simulink model "pe_pmsm_drive_project"  (R2018b)
settings: Solver=VariableStepAuto  StartTime=0.0  StopTime=0.5  FixedStep=1e-3  MaxStep=2.0E-6  RelTol=1e-6  AbsTol=1e-3  EnableMultiTasking=on
PreLoadFcn:
  | % Control parameters
  | Ts = 2e-6;   % Fundamental sample time
  | fsw = 2e3;   % Switching frequency (Hz)
  | fc = fsw*10; % Control loop frequency (Hz)
  | Tsc = 1/fc;  % Control loop sample time
  | 
  | % PMSM parameters
  | PM = 0.03; % Permanent magnet flux linkage
  | Ld = 2e-4;  % d-axis inductance
  | Lq = 2e-4;  % q-axis inductance
  | L0 = 2e-4;  % 0-axis inductance
  | Rs = 0.013; % Stator resistance
  | N = 6; % Number of pole pairs
  | J = 0.2; % Moment of inertia
  | 
  | % Operating and derived limits
  | Imax = 100;  % Max stator current (peak value)
  | Tmax = 1.5*N*PM*Imax; % Max lectromagnetic torque
  | fnom = 100;  % Nominal frequency (Hz)
  | rpm_nom = 60*fnom/N;      % Nominal rotor speed (rpm)
  | omegam_nom = 2*pi*fnom/N; % Nominal mechanical rotor speed
  | Pmax = omegam_nom*Tmax;     % Maximum power
values from neighbouring files (symbols this model uses):
  faero = 0.5*cd*frontarea*airdens.*speed.^2    [PMSM.m]    (also in PMSM_trqlimiter.m)
  rt = 3    [PMSM.m]    (also in PMSM_trqlimiter.m)
  speed = linspace(0, 60, 1000)    [PMSM.m]    (also in PMSM_trqlimiter.m)
  wheelrad = 0.3    [PMSM.m]    (also in PMSM_trqlimiter.m)
libraries: nesl_utility x12, pe_lib x10, fl_lib x8, pePmsmFieldOrientedControl x1, simulink x1
CloseFcn:
  | try
  |   clear Imax J L0 Ld Lq N PM Pmax Rs
  |   clear Tmax Ts Tsc fc fnom fsw
  |   clear omegam_nom rpm_nom tout
  | end
Description:
  | Three-Phase PMSM Drive
  | 
  | This example shows a Permanent Magnet Synchronous Machine
  | (PMSM) and inverter sized for use in a typical hybrid vehicle.
  | Here the inverter is connected directly to the vehicle battery, but
  | often there is also a DC-DC converter stage in between. The
  | model can be used to design the PMSM controller, selecting
  | architecture and gains to achieve desired performance. To check
  | the timing of IGBT turn-on and turn-off, the IGBT devices can be
  | directly replaced by more detailed device models from
  | Simscape(TM) Electronics(TM). For complete vehicle modeling, the
  | Simscape Electronics Servomotor block can be used to abstract
  | the PMSM, inverter and controller with an energy-based model.
  | The Gmin resistor provides a very small conductance to ground
  | that improves the numerical properties of the model when using
  | a variable-step solver.
  | 
  | Copyright 2014-2017 The MathWorks, Inc.
settings Model: Creator=The MathWorks, Inc.  LastModifiedBy=Giorgia
settings SolverCC: AutoScaleAbsTol=off  MaxConsecutiveMinStep=2
settings DataIOCC: LimitDataPoints=on  SaveFormat=Array
settings OptimizationCC: LifeSpan=inf
settings DebuggingCC: UnderspecifiedInitializationDetection=Classic  MergeDetectMultiDrivingBlocksExec=none  MaxConsecutiveZCsMsg=none  AllowSymbolicDim=off  LibraryContextMissingDiagnostic=none  SFUnexpectedBacktrackingDiag=warning  SFNoUnconditionalDefaultTransitionDiag=warning  SFExecutionAtInitializationDiag=none
settings HardwareCC: ProdBitPerPointer=32  ProdBitPerSizeT=32  ProdBitPerPtrDiffT=32  ProdLargestAtomicFloat=None  ProdIntDivRoundTo=Undefined  ProdEndianess=Unspecified  ProdWordSize=32  ProdHWDeviceType=32-bit Generic
settings ModelReferenceCC: PropagateSignalLabelsOutOfModel=off
settings SFSimCC: SimUseLocalCustomCode=off
settings RTWCC: RTWUseLocalCustomCode=off
settings CodeAppCC: StateflowObjectComments=on
settings GRTTargetCC: TargetLangStandard=C89/C90 (ANSI)  GeneratePreprocessorConditionals=Disable all
settings ConfigComp: CovMetricSettings=dw  CovHtmlReporting=on  CovSaveCumulativeToWorkspaceVar=on  CovSaveSingleToWorkspaceVar=on  CovShowResultsExplorer=off  CovExternalEMLEnable=off  CovSFcnEnable=off

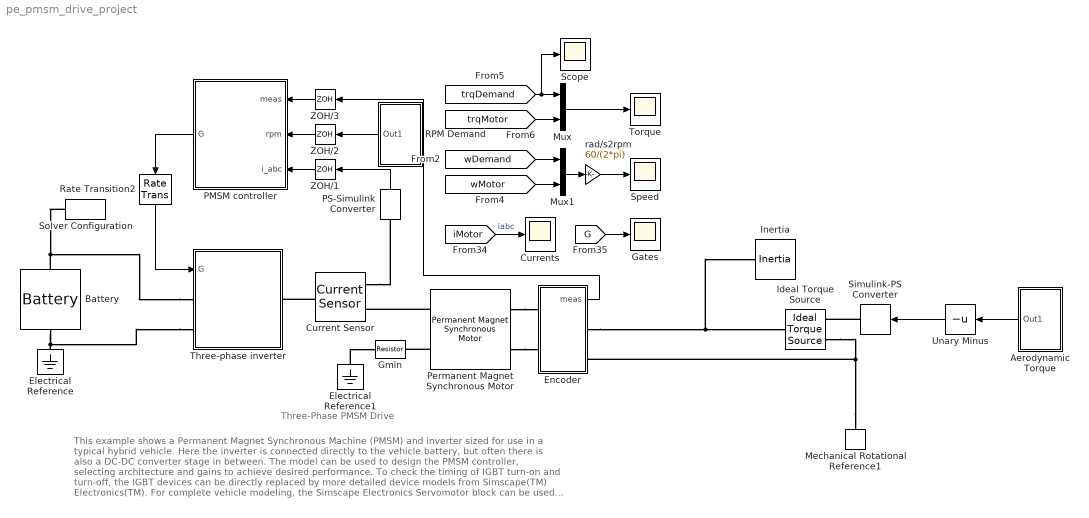
== system pe_pmsm_drive_project ==
  note: This example shows a Permanent Magnet Synchronous Machine (PMSM) and inverter sized for use in a typical hybrid vehicle.
      | Here the inverter is connected directly to the vehicle battery, but often there is also a DC-DC converter stage in between. The
      | model can be used to design the PMSM controller, selecting architecture and gains to achieve desired performance. To check
      | the timing of IGBT turn-on and turn-off, the IGBT devices can be directly replaced by more detailed device models from
      | Simscape(TM) Electronics(TM). For complete vehicle modeling, the Simscape Electronics Servomotor block can be used to
      | abstract the PMSM, inverter and controller with an energy-based model. The Gmin resistor provides a very small conductance
      | to ground that improves the numerical properties of the model when using a variable-step solver.
  note: Three-Phase PMSM Drive
  Aerodynamic Torque : Subsystem
  Battery : pe_lib/Sources/Battery  Vnom=110 V  R1=0.001 Ohm  prm_AH=1  AH=14000 hr*A  V1=470 V  AH1=5000 hr*A  prm_R2=1  R2=inf Ohm  prm_dyn=1  Rp1=0.005 Ohm  tau1=30 s  Rp2=0.005 Ohm  tau2=30 s  Rp3=0.005 Ohm  tau3=30 s  Rp4=0.005 Ohm  tau4=30 s  Rp5=0.005 Ohm  tau5=30 s  prm_fade=1  N_fade=100  AH_fade=45 hr*A  R1_fade=2.02 Ohm  V1_fade=10.35 V  i_specify=off  i_priority=None  i=0 A  i_nominal_specify=off  i_nominal_unit=A  i_nominal_value=1  v_specify=off  v_priority=None  v=0 V  v_nominal_specify=off  v_nominal_unit=V  v_nominal_value=1  charge_specify=on  charge_priority=High  charge=7000 hr*A  charge_nominal_specify=off  charge_nominal_unit=hr*A  charge_nominal_value=1  num_cycles_specify=off  num_cycles_priority=High  num_cycles=0  num_cycles_nominal_specify=off  num_cycles_nominal_unit=1  num_cycles_nominal_value=1  thermal_mass=30000 J/K  Tmeas=298.15 K  Vnom_T2=12 V  R1_T2=2.2 Ohm  V1_T2=11.4 V  R2_T2=2200 Ohm  Rp1_T2=0.005 Ohm  tau1_T2=30 s  Rp2_T2=0.005 Ohm  tau2_T2=30 s  Rp3_T2=0.005 Ohm  tau3_T2=30 s  Rp4_T2=0.005 Ohm  tau4_T2=30 s  Rp5_T2=0.005 Ohm  tau5_T2=30 s  Tmeas2=273.15 K  temperature_specify=off  temperature_priority=High  temperature=298.15 K  temperature_nominal_specify=off  temperature_nominal_unit=K  temperature_nominal_value=1
      settings: SourceProductName=Simscape Electrical  SourceProductBaseCode=PS
  Current Sensor : pe_lib/Sensors/Current Sensor
      settings: SourceProductName=Simscape Electrical  SourceProductBaseCode=PS
  Currents : Scope
  Electrical Reference : fl_lib/Electrical/Electrical Elements/Electrical Reference
      settings: SourceProductName=Foundation Library
  Electrical Reference1 : fl_lib/Electrical/Electrical Elements/Electrical Reference
      settings: SourceProductName=Foundation Library
  Encoder : Subsystem
  Gates : Scope
  Gmin : fl_lib/Electrical/Electrical Elements/Resistor  R=1e9 Ohm  i_specify=off  i_priority=High  i=0 A  i_nominal_specify=off  i_nominal_unit=A  i_nominal_value=1  v_specify=off  v_priority=High  v=0 V  v_nominal_specify=off  v_nominal_unit=V  v_nominal_value=1
      settings: SourceProductName=Foundation Library
  Ideal Torque Source : fl_lib/Mechanical/Mechanical Sources/Ideal Torque Source
  Inertia : fl_lib/Mechanical/Rotational Elements/Inertia  inertia=0.01 kg*m^2  w_specify=off  w_priority=High  w=0 rad/s  w_nominal_specify=off  w_nominal_unit=rad/s  w_nominal_value=1  t_specify=off  t_priority=None  t=0 N*m  t_nominal_specify=off  t_nominal_unit=N*m  t_nominal_value=1
  Mechanical Rotational Reference1 : fl_lib/Mechanical/Rotational Elements/Mechanical Rotational Reference
      settings: SourceProductName=Foundation Library
  Mux : Mux  Inputs=2
  Mux1 : Mux  Inputs=2
  PMSM controller : Subsystem
  PS-Simulink Converter : nesl_utility/PS-Simulink Converter  PhysicalDomain=network_engine_domain  SubClassName=ps_output  LeftPortType=input  RightPortType=output  PseudoPeriodic=off  Frequencies=[]  Unit=A  AffineConversion=off
  Permanent Magnet Synchronous Motor : pe_lib/Machines/Permanent Magnet Rotor/Permanent Magnet Synchronous Motor  nPolePairs=N  pmflux_param=1  pm_flux_linkage=PM Wb  torque_constant=0.18 N*m/A  back_emf_constant=0.18 V/(rad/s)  stator_param=1  Ld=Ld H  Lq=Lq H  L0=L0 H  Ls=0.0002 H  Lm=0.00002 H  Ms=0.00002 H  Rs=Rs Ohm  zero_sequence=pe.enum.park.zerosequence.include  J=0 kg*m^2  lam=0 N*m/(rad/s)  axes_param=1  i_d_specify=off  i_d_priority=None  i_d=0 A  i_d_nominal_specify=off  i_d_nominal_unit=A  i_d_nominal_value=1  i_q_specify=off  i_q_priority=None  i_q=0 A  i_q_nominal_specify=off  i_q_nominal_unit=A  i_q_nominal_value=1  torque_specify=off  torque_priority=None  torque=0 N*m  torque_nominal_specify=off  torque_nominal_unit=N*m  torque_nominal_value=1  angular_velocity_specify=on  angular_velocity_priority=None  angular_velocity=0 rpm  angular_velocity_nominal_specify=off  angular_velocity_nominal_unit=rpm  angular_velocity_nominal_value=1  angular_position_specify=on  angular_position_priority=High  angular_position=0 rad  angular_position_nominal_specify=off  angular_position_nominal_unit=deg  angular_position_nominal_value=1
      settings: SourceProductName=Simscape Electrical  SourceProductBaseCode=PS
  RPM Demand : Subsystem
  Rate Transition2 : RateTransition  OutPortSampleTime=Ts
  Scope : Scope
  Simulink-PS Converter : nesl_utility/Simulink-PS Converter  PhysicalDomain=network_engine_domain  SubClassName=ps_input  LeftPortType=input  RightPortType=output  PseudoPeriodic=off  Frequencies=[]  NoiseDistribution=none  NoiseParameters=[]  Unit=1  AffineConversion=off  FilteringAndDerivatives=provide  SimscapeFilterOrder=1  InputFilterTimeConstant=0.001  UdotUserProvided=0
  Solver Configuration : nesl_utility/Solver Configuration  PhysicalDomain=network_engine_domain  SubClassName=solver  LeftPortType=input  RightPortType=generic  Tones=[]  Harmonics=[]  SimulateNoise=off  Profile=off  UseLocalSampling=off  EnableSwitchedLinearOptims=on  FrequencyDomain=off  UseCCode=off  RelTol=0.001  AbsTol=1e-06  MinStep=1e-09  ToWorkspace=off  RevertToSquareIcSolve=off  NumHomotopyIterations=100  PhasorMode=off  PhasorModeNumHarmonics=1  DoDC=off  ResidualTolerance=1e-9  UseLocalSolver=on  LocalSolverChoice=NE_BACKWARD_EULER_ADVANCER  LocalSolverSampleTime=Ts  DoFixedCost=on  MaxNonlinIter=4  MaxModeIter=2  LinearAlgebra=Sparse  EquationFormulation=NE_TIME_EF  DelaysMemoryBudget=1024  AutomaticFiltering=on  FilteringTimeConstant=0.001  PartitionStorageMethod=AS_NEEDED  PartitionMemoryBudget=1024
  Speed : Scope
  Three-phase inverter : Subsystem
  Torque : Scope
  Unary Minus : UnaryMinus
  ZOH/1 : ZeroOrderHold  SampleTime=Tsc
  ZOH/2 : ZeroOrderHold  SampleTime=Tsc
  ZOH/3 : ZeroOrderHold  SampleTime=Tsc
  rad/s2rpm : Gain  Gain=60/(2*pi)
  wires:
  RPM Demand/1(Out1) -> ZOH/2/1
  PS-Simulink Converter/1 -> ZOH/1/1
  Mux1/1 -> rad/s2rpm/1
  [iMotor] -> Currents/1  "iabc"
  [G] -> Gates/1
  [wDemand] -> Mux1/1
  Mux/1 -> Torque/1
  [trqMotor] -> Mux/2
  [trqDemand] -> Scope/1, Mux/1
  Encoder/1(meas) -> ZOH/3/1
  ZOH/3/1 -> PMSM controller/1(meas)
  ZOH/2/1 -> PMSM controller/2(rpm)
  ZOH/1/1 -> PMSM controller/3(i_abc)
  Rate Transition2/1 -> Three-phase inverter/1(G)
  [wMotor] -> Mux1/2
  rad/s2rpm/1 -> Speed/1
  PMSM controller/1(G) -> Rate Transition2/1
  Aerodynamic Torque/1(Out1) -> Unary Minus/1
  Unary Minus/1 -> Simulink-PS Converter/1
  connections:
  Three-phase inverter/LConn1 -- Solver Configuration/RConn1 -- Battery/LConn1
  Permanent Magnet Synchronous Motor/RConn1 -- Encoder/LConn1
  Permanent Magnet Synchronous Motor/RConn2 -- Encoder/LConn2
  Current Sensor/LConn1 -- Three-phase inverter/RConn1
  Three-phase inverter/LConn2 -- Electrical Reference/LConn1 -- Battery/RConn1
  Permanent Magnet Synchronous Motor/LConn1 -- Current Sensor/RConn2
  Current Sensor/RConn1 -- PS-Simulink Converter/LConn1
  Permanent Magnet Synchronous Motor/LConn2 -- Gmin/RConn1
  Electrical Reference1/LConn1 -- Gmin/LConn1
  Encoder/RConn1 -- Ideal Torque Source/LConn1 -- Inertia/LConn1
  Mechanical Rotational Reference1/LConn1 -- Encoder/RConn2 -- Ideal Torque Source/RConn2
  Simulink-PS Converter/RConn1 -- Ideal Torque Source/RConn1

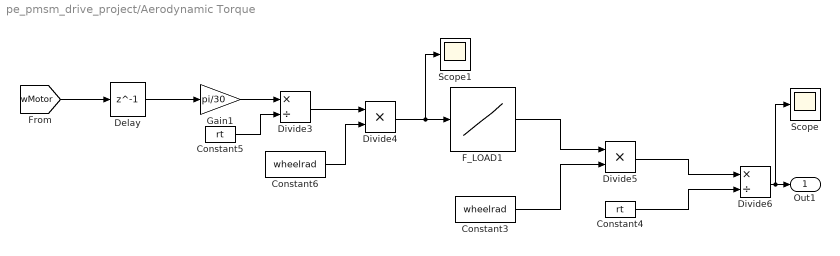
== system pe_pmsm_drive_project/Aerodynamic Torque ==
  Constant3 : Constant  Value=wheelrad
  Constant4 : Constant  Value=rt
  Constant5 : Constant  Value=rt
  Constant6 : Constant  Value=wheelrad
  Delay : Delay  DelayLength=1  InitialCondition=0
  Divide3 : Product  Inputs=*/
  Divide4 : Product  Inputs=**
  Divide5 : Product  Inputs=**
  Divide6 : Product  Inputs=*/
  F_LOAD1 : Lookup_n-D  NumberOfTableDimensions=1  BreakpointsForDimension1=speed  Table=faero  ExtrapMethod=Clip  UseLastTableValue=on  InternalRulePriority=Speed  RndMeth=Simplest  InputSameDT=on
  Gain1 : Gain  Gain=pi/30
  Scope : Scope
  Scope1 : Scope
  Out1 : Outport
  wires:
  F_LOAD1/1 -> Divide5/1
  Constant3/1 -> Divide5/2
  Divide5/1 -> Divide6/1
  Constant4/1 -> Divide6/2
  Divide6/1 -> Scope/1, Out1/1
  Constant5/1 -> Divide3/2
  Gain1/1 -> Divide3/1
  Divide3/1 -> Divide4/1
  Constant6/1 -> Divide4/2
  Divide4/1 -> Scope1/1, F_LOAD1/1
  [wMotor] -> Delay/1
  Delay/1 -> Gain1/1

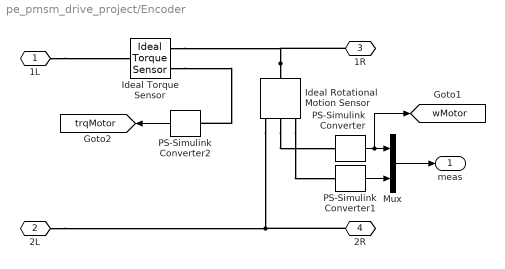
== system pe_pmsm_drive_project/Encoder ==
  Ideal Rotational Motion Sensor : fl_lib/Mechanical/Mechanical Sensors/Ideal Rotational Motion Sensor  offset=0 deg
      settings: SourceProductName=Foundation Library
  Ideal Torque Sensor : fl_lib/Mechanical/Mechanical Sensors/Ideal Torque Sensor
      settings: SourceProductName=Foundation Library
  Mux : Mux  Inputs=2
  PS-Simulink Converter : nesl_utility/PS-Simulink Converter  PhysicalDomain=network_engine_domain  SubClassName=ps_output  LeftPortType=input  RightPortType=output  PseudoPeriodic=off  Frequencies=[]  Unit=rad/s  AffineConversion=off
  PS-Simulink Converter1 : nesl_utility/PS-Simulink Converter  PhysicalDomain=network_engine_domain  SubClassName=ps_output  LeftPortType=input  RightPortType=output  PseudoPeriodic=off  Frequencies=[]  Unit=rad  AffineConversion=off
  PS-Simulink Converter2 : nesl_utility/PS-Simulink Converter  PhysicalDomain=network_engine_domain  SubClassName=ps_output  LeftPortType=input  RightPortType=output  PseudoPeriodic=off  Frequencies=[]  Unit=N*m  AffineConversion=off
  1L : PMIOPort  Side=Left
  2L : PMIOPort  Port=2  Side=Left
  1R : PMIOPort  Port=3  Side=Right
  2R : PMIOPort  Port=4  Side=Right
  meas : Outport
  tag scope: trqMotor=global, wMotor=global
  wires:
  PS-Simulink Converter2/1 -> [trqMotor]
  Mux/1 -> meas/1
  PS-Simulink Converter1/1 -> Mux/2
  PS-Simulink Converter/1 -> [wMotor], Mux/1
  connections:
  Ideal Torque Sensor/RConn2 -- PS-Simulink Converter2/LConn1
  1L/RConn1 -- Ideal Torque Sensor/LConn1
  2R/RConn1 -- 2L/RConn1 -- Ideal Rotational Motion Sensor/RConn1
  Ideal Rotational Motion Sensor/LConn1 -- 1R/RConn1 -- Ideal Torque Sensor/RConn1
  Ideal Rotational Motion Sensor/RConn2 -- PS-Simulink Converter/LConn1
  Ideal Rotational Motion Sensor/RConn3 -- PS-Simulink Converter1/LConn1

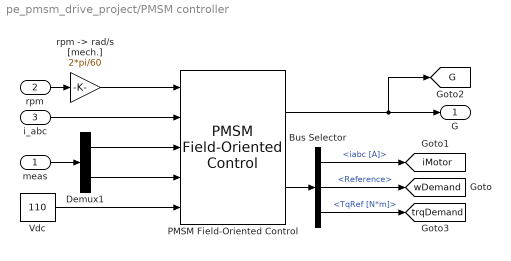
== system pe_pmsm_drive_project/PMSM controller ==
  meas : Inport
  rpm : Inport  Port=2
  i_abc : Inport  Port=3
  Bus Selector : BusSelector  OutputSignals=iabc [A],Reference,TqRef [N*m]
  Demux1 : Demux  Outputs=2
  PMSM Field-Oriented Control : pePmsmFieldOrientedControl/PMSM Field-Oriented Control  CtrlMode=Velocity control  Vnom=110  Pmax=Pmax  Tmax=Tmax*1.5  p=N  Vdc_on=10  Ts=Ts  Tsc=Tsc  CtrlType=PI control  Kp_w=6  Ki_w=200  Kv_w=1  Kaw_w=1000  RefType=Zero d-axis control  rpmVec=[0, 3000]  TqVec=[-100, 0, 100]  VdcVec=[300, 350]  idMatrix=zeros(2,3,2)  iqMatrix=zeros(2,3,2)  psim=PM  Ld=0.00024  Lq=0.00029  Rs=0.01  AxisAlignment=Q-axis  Kp_id=0.1  Ki_id=10  Kaw_id=1000  Kp_iq=0.1  Ki_iq=10  Kaw_iq=1000  AxisPrio=Q-axis  ActZC=off  ActFF=on  ParamTypeFF=Constant parameters  LdFF=Ld  LqFF=Lq  psimFF=PM  idVect=[-200, 0, 200]  iqVect=[-200, 0, 200]  LdMatrix=0.0002 * ones(3, 3)  LqMatrix=0.0002 * ones(3, 3)  psimMatrix=0.04 * ones(3, 3)  CPWMMode=SPWM: sinusoidal PWM  fsw=fsw
      settings: SamplingMode=Natural
  Vdc : Constant  Value=110  SampleTime=Tsc
  "rpm -> rad/s [mech.]" : Gain  Gain=2*pi/60
  G : Outport
  tag scope: G=global, iMotor=global, trqDemand=global, wDemand=global
  wires:
  PMSM Field-Oriented Control/1 -> G/1, [G]
  Vdc/1 -> PMSM Field-Oriented Control/5
  PMSM Field-Oriented Control/2 -> Bus Selector/1
  i_abc/1 -> PMSM Field-Oriented Control/2
  meas/1 -> Demux1/1
  Demux1/1 -> PMSM Field-Oriented Control/3
  Demux1/2 -> PMSM Field-Oriented Control/4
  Bus Selector/1 -> [iMotor]  "<iabc [A]>"
  Bus Selector/2 -> [wDemand]  "<Reference>"
  Bus Selector/3 -> [trqDemand]  "<TqRef [N*m]>"
  rpm/1 -> "rpm -> rad/s [mech.]"/1
  "rpm -> rad/s [mech.]"/1 -> PMSM Field-Oriented Control/1

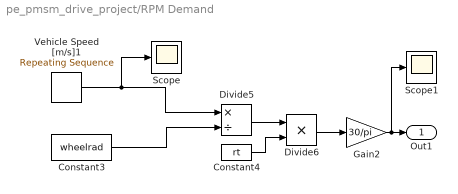
== system pe_pmsm_drive_project/RPM Demand ==
  Constant3 : Constant  Value=wheelrad
  Constant4 : Constant  Value=rt
  Divide5 : Product  Inputs=*/
  Divide6 : Product  Inputs=**
  Gain2 : Gain  Gain=30/pi
  Scope : Scope
  Scope1 : Scope
  Vehicle Speed [m/s]1 : simulink/Sources/Repeating Sequence  rep_seq_t=time  rep_seq_y=vehiclespeed
  Out1 : Outport
  wires:
  Vehicle Speed [m/s]1/1 -> Scope/1, Divide5/1
  Constant4/1 -> Divide6/2
  Divide6/1 -> Gain2/1
  Divide5/1 -> Divide6/1
  Constant3/1 -> Divide5/2
  Gain2/1 -> Scope1/1, Out1/1

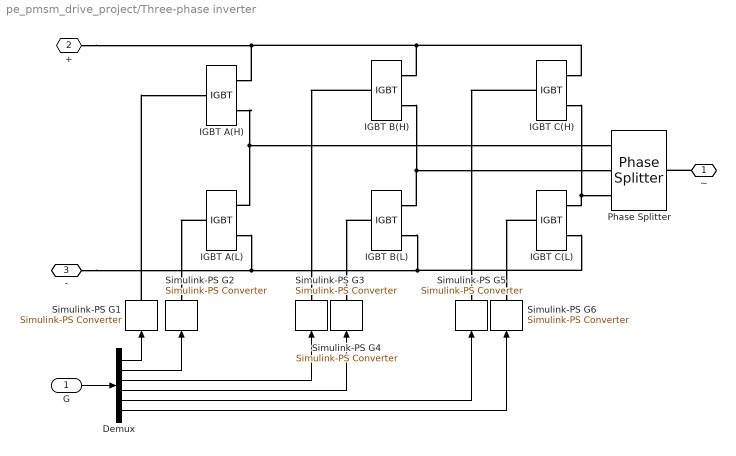
== system pe_pmsm_drive_project/Three-phase inverter ==
  G : Inport
  Demux : Demux  Outputs=6
  IGBT A(H) : pe_lib/Semiconductors/Fundamental Components/IGBT  Vf=0.8 V  Ron=0.001 Ohm  Goff=1e-5 S  Vth=0.5 V  diode_param=2  diode_Vf=0.8 V  diode_Ron=0.001 Ohm  diode_Goff=1e-5 S  diode_C=5e-8 F  diode_iRM=-235 A  diode_iF=300 A  diode_idot=-50 A/us  diode_trr_param=1  diode_trr_factor=3  diode_trr=15 us  diode_Qrr=1.5e+3 s*uA  thermal_loss_option=1  Voff=300 V  Tau=0.1 s  Tj=[ 298.15 398.15 ] K  Iout_scalar=600 A  Eon_scalar=0.02286 J  Eoff_scalar=0.01714 J  Von_scalar=2.7 V  Iout_data=[ 0 10 50 100 200 400 600 ] A  Eon_data=[ 0 2.9e-4 0.00143 0.00286 0.00571 0.01314 0.02286; 0 5.7e-4 0.00263 0.00514 0.01029 0.02057 0.03029 ] J  Eoff_data=[ 0 2.1e-4 0.00107 0.00214 0.00429 0.009859999999999999 0.01714; 0 4.3e-4 0.00197 0.00386 0.00771 0.01543 0.02271 ] J  Von_data=[ 0 1.1 1.3 1.45 1.75 2.25 2.7; 0 1 1.15 1.35 1.7 2.35 3 ] V
      settings: SourceProductName=Simscape Electrical  SourceProductBaseCode=PS
  IGBT A(L) : pe_lib/Semiconductors/Fundamental Components/IGBT  Vf=0.8 V  Ron=0.001 Ohm  Goff=1e-5 S  Vth=0.5 V  diode_param=2  diode_Vf=0.8 V  diode_Ron=0.001 Ohm  diode_Goff=1e-5 S  diode_C=5e-8 F  diode_iRM=-235 A  diode_iF=300 A  diode_idot=-50 A/us  diode_trr_param=1  diode_trr_factor=3  diode_trr=15 us  diode_Qrr=1.5e+3 s*uA  thermal_loss_option=1  Voff=300 V  Tau=0.1 s  Tj=[ 298.15 398.15 ] K  Iout_scalar=600 A  Eon_scalar=0.02286 J  Eoff_scalar=0.01714 J  Von_scalar=2.7 V  Iout_data=[ 0 10 50 100 200 400 600 ] A  Eon_data=[ 0 2.9e-4 0.00143 0.00286 0.00571 0.01314 0.02286; 0 5.7e-4 0.00263 0.00514 0.01029 0.02057 0.03029 ] J  Eoff_data=[ 0 2.1e-4 0.00107 0.00214 0.00429 0.009859999999999999 0.01714; 0 4.3e-4 0.00197 0.00386 0.00771 0.01543 0.02271 ] J  Von_data=[ 0 1.1 1.3 1.45 1.75 2.25 2.7; 0 1 1.15 1.35 1.7 2.35 3 ] V
      settings: SourceProductName=Simscape Electrical  SourceProductBaseCode=PS
  IGBT B(H) : pe_lib/Semiconductors/Fundamental Components/IGBT  Vf=0.8 V  Ron=0.001 Ohm  Goff=1e-5 S  Vth=0.5 V  diode_param=2  diode_Vf=0.8 V  diode_Ron=0.001 Ohm  diode_Goff=1e-5 S  diode_C=5e-8 F  diode_iRM=-235 A  diode_iF=300 A  diode_idot=-50 A/us  diode_trr_param=1  diode_trr_factor=3  diode_trr=15 us  diode_Qrr=1.5e+3 s*uA  thermal_loss_option=1  Voff=300 V  Tau=0.1 s  Tj=[ 298.15 398.15 ] K  Iout_scalar=600 A  Eon_scalar=0.02286 J  Eoff_scalar=0.01714 J  Von_scalar=2.7 V  Iout_data=[ 0 10 50 100 200 400 600 ] A  Eon_data=[ 0 2.9e-4 0.00143 0.00286 0.00571 0.01314 0.02286; 0 5.7e-4 0.00263 0.00514 0.01029 0.02057 0.03029 ] J  Eoff_data=[ 0 2.1e-4 0.00107 0.00214 0.00429 0.009859999999999999 0.01714; 0 4.3e-4 0.00197 0.00386 0.00771 0.01543 0.02271 ] J  Von_data=[ 0 1.1 1.3 1.45 1.75 2.25 2.7; 0 1 1.15 1.35 1.7 2.35 3 ] V
      settings: SourceProductName=Simscape Electrical  SourceProductBaseCode=PS
  IGBT B(L) : pe_lib/Semiconductors/Fundamental Components/IGBT  Vf=0.8 V  Ron=0.001 Ohm  Goff=1e-5 S  Vth=0.5 V  diode_param=2  diode_Vf=0.8 V  diode_Ron=0.001 Ohm  diode_Goff=1e-5 S  diode_C=5e-8 F  diode_iRM=-235 A  diode_iF=300 A  diode_idot=-50 A/us  diode_trr_param=1  diode_trr_factor=3  diode_trr=15 us  diode_Qrr=1.5e+3 s*uA  thermal_loss_option=1  Voff=300 V  Tau=0.1 s  Tj=[ 298.15 398.15 ] K  Iout_scalar=600 A  Eon_scalar=0.02286 J  Eoff_scalar=0.01714 J  Von_scalar=2.7 V  Iout_data=[ 0 10 50 100 200 400 600 ] A  Eon_data=[ 0 2.9e-4 0.00143 0.00286 0.00571 0.01314 0.02286; 0 5.7e-4 0.00263 0.00514 0.01029 0.02057 0.03029 ] J  Eoff_data=[ 0 2.1e-4 0.00107 0.00214 0.00429 0.009859999999999999 0.01714; 0 4.3e-4 0.00197 0.00386 0.00771 0.01543 0.02271 ] J  Von_data=[ 0 1.1 1.3 1.45 1.75 2.25 2.7; 0 1 1.15 1.35 1.7 2.35 3 ] V
      settings: SourceProductName=Simscape Electrical  SourceProductBaseCode=PS
  IGBT C(H) : pe_lib/Semiconductors/Fundamental Components/IGBT  Vf=0.8 V  Ron=0.001 Ohm  Goff=1e-5 S  Vth=0.5 V  diode_param=2  diode_Vf=0.8 V  diode_Ron=0.001 Ohm  diode_Goff=1e-5 S  diode_C=5e-8 F  diode_iRM=-235 A  diode_iF=300 A  diode_idot=-50 A/us  diode_trr_param=1  diode_trr_factor=3  diode_trr=15 us  diode_Qrr=1.5e+3 s*uA  thermal_loss_option=1  Voff=300 V  Tau=0.1 s  Tj=[ 298.15 398.15 ] K  Iout_scalar=600 A  Eon_scalar=0.02286 J  Eoff_scalar=0.01714 J  Von_scalar=2.7 V  Iout_data=[ 0 10 50 100 200 400 600 ] A  Eon_data=[ 0 2.9e-4 0.00143 0.00286 0.00571 0.01314 0.02286; 0 5.7e-4 0.00263 0.00514 0.01029 0.02057 0.03029 ] J  Eoff_data=[ 0 2.1e-4 0.00107 0.00214 0.00429 0.009859999999999999 0.01714; 0 4.3e-4 0.00197 0.00386 0.00771 0.01543 0.02271 ] J  Von_data=[ 0 1.1 1.3 1.45 1.75 2.25 2.7; 0 1 1.15 1.35 1.7 2.35 3 ] V
      settings: SourceProductName=Simscape Electrical  SourceProductBaseCode=PS
  IGBT C(L) : pe_lib/Semiconductors/Fundamental Components/IGBT  Vf=0.8 V  Ron=0.001 Ohm  Goff=1e-5 S  Vth=0.5 V  diode_param=2  diode_Vf=0.8 V  diode_Ron=0.001 Ohm  diode_Goff=1e-5 S  diode_C=5e-8 F  diode_iRM=-235 A  diode_iF=300 A  diode_idot=-50 A/us  diode_trr_param=1  diode_trr_factor=3  diode_trr=15 us  diode_Qrr=1.5e+3 s*uA  thermal_loss_option=1  Voff=300 V  Tau=0.1 s  Tj=[ 298.15 398.15 ] K  Iout_scalar=600 A  Eon_scalar=0.02286 J  Eoff_scalar=0.01714 J  Von_scalar=2.7 V  Iout_data=[ 0 10 50 100 200 400 600 ] A  Eon_data=[ 0 2.9e-4 0.00143 0.00286 0.00571 0.01314 0.02286; 0 5.7e-4 0.00263 0.00514 0.01029 0.02057 0.03029 ] J  Eoff_data=[ 0 2.1e-4 0.00107 0.00214 0.00429 0.009859999999999999 0.01714; 0 4.3e-4 0.00197 0.00386 0.00771 0.01543 0.02271 ] J  Von_data=[ 0 1.1 1.3 1.45 1.75 2.25 2.7; 0 1 1.15 1.35 1.7 2.35 3 ] V
      settings: SourceProductName=Simscape Electrical  SourceProductBaseCode=PS
  Phase Splitter : pe_lib/Connections/Phase Splitter
      settings: SourceProductName=Simscape Electrical  SourceProductBaseCode=PS
  Simulink-PS G{1..6} (6 alike) : nesl_utility/Simulink-PS Converter  PhysicalDomain=network_engine_domain  SubClassName=ps_input  LeftPortType=input  RightPortType=output  PseudoPeriodic=off  Frequencies=[]  NoiseDistribution=none  NoiseParameters=[]  Unit=1  AffineConversion=off  FilteringAndDerivatives=zero  SimscapeFilterOrder=1  InputFilterTimeConstant=1e-6  UdotUserProvided=0
  ~ : PMIOPort  Tag=PMCPort  Side=Right
  + : PMIOPort  Tag=PMCPort  Port=2  Side=Left
  - : PMIOPort  Tag=PMCPort  Port=3  Side=Left
  wires:
  Demux/6 -> Simulink-PS G6/1
  Demux/5 -> Simulink-PS G5/1
  Demux/4 -> Simulink-PS G4/1
  Demux/3 -> Simulink-PS G3/1
  Demux/2 -> Simulink-PS G2/1
  G/1 -> Demux/1
  Demux/1 -> Simulink-PS G1/1
  connections:
  IGBT C(L)/LConn1 -- Simulink-PS G6/RConn1
  IGBT C(H)/LConn1 -- Simulink-PS G5/RConn1
  IGBT B(L)/LConn1 -- Simulink-PS G4/RConn1
  IGBT B(H)/LConn1 -- Simulink-PS G3/RConn1
  IGBT A(L)/LConn1 -- Simulink-PS G2/RConn1
  -/RConn1 -- IGBT A(L)/RConn2 -- IGBT C(L)/RConn2 -- IGBT B(L)/RConn2
  IGBT A(H)/RConn2 -- IGBT A(L)/RConn1 -- Phase Splitter/RConn1
  IGBT B(L)/RConn1 -- IGBT B(H)/RConn2 -- Phase Splitter/RConn2
  IGBT C(L)/RConn1 -- IGBT C(H)/RConn2 -- Phase Splitter/RConn3
  +/RConn1 -- IGBT A(H)/RConn1 -- IGBT C(H)/RConn1 -- IGBT B(H)/RConn1
  ~/RConn1 -- Phase Splitter/LConn1
  Simulink-PS G1/RConn1 -- IGBT A(H)/LConn1
